simulink model "ModeAdjust"  (R2018b)
settings: Solver=FixedStepDiscrete  StartTime=0.0  StopTime=inf  FixedStep=0.01  RelTol=1e-3
undefined symbols (not defined in the file or in its folder): IfKeSMSbSeatMovBkRclnEnable_Val, IfKeSMSbSeatMovFrwdBkwdEnable_Val, IfKeSMSbSeatMovFtrstEnable_Val, IfKeSMSbSeatMovHdrstFrwdBkwdEnable_Val, IfKeSMSbSeatMovHdUpwdDnwdEnable_Val, IfKeSMSbSeatMovLgrstEnable_Val, IfKeSMSbSeatMovLtwdRtwdEnable_Val, IfVeSMSeStNumConfig, KeSMSbArmscreenMovEnable_Val, KeSMSbSeatMovLgrstExpdEnable_Val, KeSMSuFirstRwStBackPosDelta_Val, KeSMSuFirstRwStBackPosTolr_Val, KeSMSuFirstRwStCushFrntPosDelta_Val, KeSMSuFirstRwStCushFrntPosTolr_Val, KeSMSuFirstRwStCushRePosDelta_Val, KeSMSuFirstRwStCushRePosTolr_Val, KeSMSuFirstRwStFootrestPosDelta_Val, KeSMSuFirstRwStFootrestPosTolr_Val, KeSMSuFirstRwStFwdBkwdPosDelta_Val, KeSMSuFirstRwStFwdBkwdPosTolr_Val, KeSMSuMdMotFinshdTm_Val, KeSMSuMdRetryTm1_Val, KeSMSuModeReqDurgTm_Val, KeSMSuSecRwStArmTochPosDelta_Val, KeSMSuSecRwStArmTochPosTolr_Val, KeSMSuSecRwStBackPosDelta_Val, KeSMSuSecRwStBackPosTolr_Val, KeSMSuSecRwStFtrstUpwdDnwdPosDelta_Val, KeSMSuSecRwStFtrstUpwdDnwdPosTolr_Val, KeSMSuSecRwStFwdBkwdPosDelta_Val, KeSMSuSecRwStFwdBkwdPosTolr_Val, KeSMSuSecRwStHeadrestFwdBkwdPosDelta_Val, KeSMSuSecRwStHeadrestFwdBkwdPosTolr_Val, KeSMSuSecRwStHeadrestUpwdDwnwdPosDelta_Val, KeSMSuSecRwStHeadrestUpwdDwnwdPosTolr_Val, KeSMSuSecRwStLegrestInOutPosDelta_Val, KeSMSuSecRwStLegrestInOutPosTolr_Val, KeSMSuSecRwStLegrestUpwdDwnwdPosDelta_Val, KeSMSuSecRwStLegrestUpwdDwnwdPosTolr_Val, KeSMSuSecRwStLwdRwdPosDelta_Val, KeSMSuSecRwStLwdRwdPosTolr_Val, KeSMSuSecRwStVIPFtrstRefAngle_Val, KeSMSuThirdRwStFwdBkwdPosDelta_Val, KeSMSuThirdRwStFwdBkwdPosTolr_Val, KeSMSuThrdRwCushFoldPosDelta_Val, KeSMSuThrdRwCushFoldPosTolr_Val, KeSMSuThrdRwStBackPosDelta_Val, KeSMSuThrdRwStBackPosTolr_Val, KeSMSw4SLegrstCloseMdSecRwLtStFtrstUpwdDnwdPos_Val, KeSMSw4SLegrstCloseMdSecRwLtStFtrstUpwdDnwdPosMax_Val, KeSMSw4SLegrstCloseMdSecRwLtStFtrstUpwdDnwdPosMin_Val, KeSMSw4SLegrstCloseMdSecRwLtStLgrstOtwdInwdPos_Val, KeSMSw4SLegrstCloseMdSecRwLtStLgrstOtwdInwdPosMax_Val, KeSMSw4SLegrstCloseMdSecRwLtStLgrstOtwdInwdPosMin_Val, KeSMSw4SLegrstCloseMdSecRwLtStLgrstUpwdDnwdPos_Val, KeSMSw4SLegrstCloseMdSecRwLtStLgrstUpwdDnwdPosMax_Val, KeSMSw4SLegrstCloseMdSecRwLtStLgrstUpwdDnwdPosMin_Val, KeSMSw4SLegrstCloseMdSecRwRtStFtrstUpwdDnwdPos_Val, KeSMSw4SLegrstCloseMdSecRwRtStFtrstUpwdDnwdPosMax_Val, KeSMSw4SLegrstCloseMdSecRwRtStFtrstUpwdDnwdPosMin_Val ... (+1138)
libraries: Lib x401
(part 8 of 35)

== system ModeAdjust/ModeAdjustRunnable_sys/ModeAdjust/LgrstCloseR ==
  note: Change Request 179276
      | 复位模式头枕上下移动到第一步，第一步直接控制靠背、头枕上下、腿托系统同时运动，
      | 当腿托系统运动完成后进行头枕前后运动
  SecRwLtStsPoss : Inport
  SecRwLtStPossV : Inport  Port=2
  Recovery_Mod_Left : Inport  Port=3
  ModeStCalib : Inport  Port=4
  StConfig : Inport  Port=5
  SecRwLtStsPoss4s : Inport  Port=6
  SecRwLtStPossV4s : Inport  Port=7
  StConfig4s : Inport  Port=8
  isLfRecoveryArrivedAtTargetPos : Inport  Port=9
  Enable : EnablePort  StatesWhenEnabling=reset
  Bus Creator1 : BusCreator  Inputs=2
  Bus Selector : BusSelector  OutputSignals=Calib_Drv,Calib_Pass,Calib_2L,Calib_2R,Calib_3L,Calib_3R,Calib_2L4s,Calib_2R4s
  Bus Selector1 : BusSelector  OutputSignals=DrvStConfig,PassStConfig,SecRwLtStConfig,SecRwRtStConfig,ThdRwLtStConfig,ThdRwRtStConfig
  Bus Selector2 : BusSelector  OutputSignals=SecRwLtStConfig,SecRwRtStConfig
  Bus Selector3 : BusSelector  OutputSignals=IfVeSMSuSecRwRtStBkReclnUpwdDnwdPos_Val_read,IfVeSMSuSecRwRtStFrwdBkwdPos_Val_read,IfVeSMSuSecRwRtStHPassStUpwdDnwdPos_Val_read,IfVeSMSuSecRwRtStLgrstUpwdDnwdPos_Val_read,IfVeSMSuSecRwRtStLtwdRtwdPos_Val_read,SecRwRtStArmScrnPos_Val_read
  Bus Selector4 : BusSelector  OutputSignals=IfVeSMSuSecRwRtStBkReclnUpwdDnwdPosV_Val_read,IfVeSMSuSecRwRtStFrwdBkwdPosV_Val_read,IfVeSMSuSecRwRtStHPassStUpwdDnwdPosV_Val_read,IfVeSMSuSecRwRtStLgrstUpwdDnwdPosV_Val_read,IfVeSMSuSecRwRtStLtwdRtwdPosV_Val_read,SecRwRtStArmScrnPosV_Val_read
  Bus Selector5 : BusSelector  OutputSignals=IfVeSMSuSecRwRtStLgrstOtwdInwdPos_Val_read,IfVeSMSuRrRtStFtUpwdDnwdPos_Val_read,IfVeSMSuSecRwRtStHdrstFrwdBkwdPos_Val_read
  Bus Selector6 : BusSelector  OutputSignals=IfVeSMSuSecRwRtStLgrstOtwdInwdPosV_Val_read,IfVeSMSuRrRtStFtUpwdDnwdPosV_Val_read
  Chart : Stateflow chart  TreatAsAtomicUnit=on
  Chart1 : Stateflow chart  TreatAsAtomicUnit=on
  Logical Operator1 : Logic  Operator=NOT  AllPortsSameDT=off  OutDataTypeStr=boolean
  Logical Operator2 : Logic  Inputs=3  AllPortsSameDT=off  OutDataTypeStr=boolean
  Logical Operator3 : Logic  Operator=OR  AllPortsSameDT=off  OutDataTypeStr=boolean
  PA_KeSMSuSecRwStFtrstUpwdDnwdPosDelta_Val : Constant  Value=KeSMSuSecRwStFtrstUpwdDnwdPosDelta_Val
  PA_KeSMSuSecRwStLegrestInOutPosDelta_Val : Constant  Value=KeSMSuSecRwStLegrestInOutPosDelta_Val
  PA_KeSMSw4SSecRwLtStLgrstOtwdInwdClosePos1_Val : Constant  Value=KeSMSw4SSecRwLtStLgrstOtwdInwdClosePos1_Val
  PA_KeSMSw4SSecRwLtStLgrstUpwdDnwdClosePos1_Val : Constant  Value=KeSMSw4SSecRwLtStLgrstUpwdDnwdClosePos1_Val
  PA_KeSMSw4SSecRwLtStLgrstUpwdDnwdClosePos2_Val : Constant  Value=KeSMSw4SSecRwLtStLgrstUpwdDnwdClosePos2_Val
  R2Lt : Subsystem
  VIP_TrigJudg : Lib/VIP_TrigJudg  SystemSampleTime=-1
  R2Lt_TrgtPoss : Outport  VectorParamsAs1DForOutWhenUnconnected=on
  IfVeSMSuSecRwLtStRclCmdSrv_Val_writeRec : Outport  Port=2
  isAcsMdFeedBackNew_LyL : Outport  Port=3
  R2Lt_TrgtPoss_2 : Outport  Port=4  VectorParamsAs1DForOutWhenUnconnected=on
  wires:
  Logical Operator3/1 -> Chart1/1(Left_Done)
  R2Lt/2(IfVeSMSuSecRwLtStRclCmdSrv_Val_writeRaw) -> [IfVeSMSuSecRwLtStRclCmdSrv_Val_writeRaw]
  [IfVeSMSuSecRwLtStRclCmdSrv_Val_writeRaw] -> Chart1/2(IfVeSMSuSecRwLtStRclCmdSrv_Val_writeRaw)
  Recovery_Mod_Left/1 -> [Recovery_Mod_Left]
  VIP_TrigJudg/1 -> [EZE_TrigL]
  [EZE_TrigL] -> R2Lt/1(Mode_Trig)
  R2Lt/1(R2Lt_TrgtPoss) -> R2Lt_TrgtPoss/1
  SecRwLtStsPoss/1 -> R2Lt/2(SecRwLtStsPoss), [Pos]
  SecRwLtStPossV/1 -> R2Lt/3(SecRwLtStPossV), [PosV]
  [Recv_L_DoneOK] -> Chart1/3(Md_L_DoneOkRaw)
  [Recv_L_DoneFailed] -> Chart1/4(Md_L_DoneFailedRaw)
  Chart1/2(Md_L_DoneOk) -> [Ly_L_DoneOK]
  Chart1/3(Md_L_DoneFailed) -> [Ly_L_DoneFailed]
  Chart1/1(IfVeSMSuSecRwLtStRclCmdSrv_Val_write) -> IfVeSMSuSecRwLtStRclCmdSrv_Val_writeRec/1  "IfVeSMSuSecRwLtStRclCmdSrv_Val_write"
  Bus Selector/2 -> [ModeStCalib_Pass]  "<Calib_Pass>"
  Bus Selector/5 -> [ModeStCalib_3L]  "<Calib_3L>"
  Bus Selector/3 -> [ModeStCalib_2L]  "<Calib_2L>"
  Bus Selector/1 -> [ModeStCalib_Drv]  "<Calib_Drv>"
  Bus Selector/6 -> [ModeStCalib_3R]  "<Calib_3R>"
  Bus Selector/4 -> [ModeStCalib_2R]  "<Calib_2R>"
  ModeStCalib/1 -> Bus Selector/1
  [ModeStCalib_2R4s] -> R2Lt/4(ModeStCalib_2L)
  [Recovery_Mod_Left] -> VIP_TrigJudg/1
  Bus Creator1/1 -> isAcsMdFeedBackNew_LyL/1
  [Ly_L_DoneOK] -> Bus Creator1/1  "isLgrstCloseRDoneOK"
  [Ly_L_DoneFailed] -> Bus Creator1/2  "isLgrstCloseRDoneFailed"
  Bus Selector1/6 -> [ThdRwRtStConfig]  "<ThdRwRtStConfig>"
  Bus Selector1/1 -> [DrvStConfig]  "<DrvStConfig>"
  Bus Selector1/3 -> [SecRwLtStConfig]  "<SecRwLtStConfig>"
  Bus Selector1/4 -> [SecRwRtStConfig]  "<SecRwRtStConfig>"
  StConfig/1 -> Bus Selector1/1
  Bus Selector1/2 -> [PassStConfig]  "<PassStConfig>"
  Bus Selector1/5 -> [ThdRwLtStConfig]  "<ThdRwLtStConfig>"
  [SecRwLtStConfig] -> R2Lt/5(StConfig)
  Bus Selector/8 -> [ModeStCalib_2R4s]  "<Calib_2R4s>"
  Bus Selector/7 -> [ModeStCalib_2L4s]  "<Calib_2L4s>"
  SecRwLtStsPoss4s/1 -> [Pos4s], R2Lt/6(SecRwLtStsPoss4s)
  SecRwLtStPossV4s/1 -> R2Lt/7(SecRwLtStPossV4s), [PosV4s]
  StConfig4s/1 -> Bus Selector2/1
  Bus Selector2/1 -> [SecRwLtStConfig4s]  "<SecRwLtStConfig>"
  Bus Selector2/2 -> [SecRwRtStConfig4s]  "<SecRwRtStConfig>"
  [SecRwLtStConfig4s] -> R2Lt/8(StConfig4s)
  [PosV] -> Bus Selector4/1
  Bus Selector4/6 -> [R2LtStArmScrnPosV]  "<SecRwRtStArmScrnPosV_Val_read>"
  Bus Selector3/6 -> [R2LtStArmScrnPos]  "<SecRwRtStArmScrnPos_Val_read>"
  Bus Selector4/5 -> [SecRwLtStLtwdRtwdPosV]  "<IfVeSMSuSecRwRtStLtwdRtwdPosV_Val_read>"
  Bus Selector3/4 -> [SecRwLtStLgrstUpwdDnwdPos]  "<IfVeSMSuSecRwRtStLgrstUpwdDnwdPos_Val_read>"
  Bus Selector3/1 -> [SecRwLtStBkReclnUpwdDnwdPos]  "<IfVeSMSuSecRwRtStBkReclnUpwdDnwdPos_Val_read>"
  Bus Selector3/2 -> [SecRwLtStFrwdBkwdPos]  "<IfVeSMSuSecRwRtStFrwdBkwdPos_Val_read>"
  Bus Selector4/2 -> [SecRwLtStFrwdBkwdPosV]  "<IfVeSMSuSecRwRtStFrwdBkwdPosV_Val_read>"
  Bus Selector4/4 -> [SecRwLtStLgrstUpwdDnwdPosV]  "<IfVeSMSuSecRwRtStLgrstUpwdDnwdPosV_Val_read>"
  Bus Selector3/3 -> [SecRwLtStHPassStUpwdDnwdPos]  "<IfVeSMSuSecRwRtStHPassStUpwdDnwdPos_Val_read>"
  [Pos] -> Bus Selector3/1
  Bus Selector3/5 -> [SecRwLtStLtwdRtwdPos]  "<IfVeSMSuSecRwRtStLtwdRtwdPos_Val_read>"
  Bus Selector4/3 -> [SecRwLtStHPassStUpwdDnwdPosV]  "<IfVeSMSuSecRwRtStHPassStUpwdDnwdPosV_Val_read>"
  Bus Selector4/1 -> [SecRwLtStBkReclnUpwdDnwdPosV]  "<IfVeSMSuSecRwRtStBkReclnUpwdDnwdPosV_Val_read>"
  Bus Selector6/1 -> [SecRwLtStLgrstOtwdInwdPosV]  "<IfVeSMSuSecRwRtStLgrstOtwdInwdPosV_Val_read>"
  [Pos4s] -> Bus Selector5/1
  Bus Selector6/2 -> [RrLtStFtUpwdDnwdPosV]  "<IfVeSMSuRrRtStFtUpwdDnwdPosV_Val_read>"
  [PosV4s] -> Bus Selector6/1
  Bus Selector5/1 -> [SecRwLtStLgrstOtwdInwdPos]  "<IfVeSMSuSecRwRtStLgrstOtwdInwdPos_Val_read>"
  Bus Selector5/2 -> [RrLtStFtUpwdDnwdPos]  "<IfVeSMSuRrRtStFtUpwdDnwdPos_Val_read>"
  [SecRwLtStLgrstUpwdDnwdPos] -> Chart/1(downpos)
  [lgrstStep1_done] -> Chart/7(Step1done)
  [lgrstStep1_ini] -> Chart/10(Step1_ini)
  [lgrstStep2_ini] -> Chart/11(Step2_ini)
  [lgrstStep3_ini] -> Chart/12(Step3_ini)
  [lgrstStep2_done] -> Chart/8(Step2done)
  Chart/1(StepEn_LgrstStep1) -> [StepEn_LgrstStep1]
  Chart/2(StepEn_LgrstStep2) -> [StepEn_LgrstStep2]
  Chart/3(StepEn_LgrstStep3) -> [StepEn_LgrstStep3]
  R2Lt/9(R2Lt_TrgtPoss_2) -> R2Lt_TrgtPoss_2/1
  [lgrstStep3_done] -> Chart/9(Step3done)
  PA_KeSMSw4SSecRwLtStLgrstOtwdInwdClosePos1_Val/1 -> [CloseOtwdPos1]
  PA_KeSMSw4SSecRwLtStLgrstUpwdDnwdClosePos2_Val/1 -> [CloseDnwdPos2]
  PA_KeSMSw4SSecRwLtStLgrstUpwdDnwdClosePos1_Val/1 -> [CloseDnwdPos1]
  [CloseDnwdPos2] -> Chart/5(closedownpos2)
  [CloseDnwdPos1] -> Chart/4(closedownpos1)
  [CloseOtwdPos1] -> Chart/6(closeOtpos1)
  [RrLtStFtUpwdDnwdPos] -> Chart/3(Ftpos)
  [SecRwLtStLgrstOtwdInwdPos] -> Chart/2(Otpos)
  [StepEn_LgrstStep1] -> R2Lt/11(StepEn_LgrstStep3)
  [StepEn_LgrstStep3] -> R2Lt/10(StepEn_LgrstStep2)
  [StepEn_LgrstStep2] -> R2Lt/9(StepEn_LgrstStep1)
  PA_KeSMSuSecRwStFtrstUpwdDnwdPosDelta_Val/1 -> [KeSMSuSecRwStFtrstUpwdDnwdPosDelta_Val]
  [KeSMSuSecRwStFtrstUpwdDnwdPosDelta_Val] -> Chart/13(FtposDelta)
  R2Lt/6(lgrstStep1_done) -> [lgrstStep2_done]
  R2Lt/8(lgrstStep3_done) -> [lgrstStep1_done]
  R2Lt/7(lgrstStep2_done) -> [lgrstStep3_done]
  R2Lt/3(lgrstUpwd_ini) -> [lgrstStep2_ini]
  R2Lt/5(lgrstOtwd_ini) -> [lgrstStep1_ini]
  R2Lt/4(lgrstFtUpwd_ini) -> [lgrstStep3_ini]
  Logical Operator1/1 -> [Recv_L_DoneFailed]
  isLfRecoveryArrivedAtTargetPos/1 -> [Recv_L_DoneOK], Logical Operator1/1
  Bus Selector5/3 -> [SecRwLtStHdrstFrwdBkwdPos]  "<IfVeSMSuSecRwRtStHdrstFrwdBkwdPos_Val_read>"
  PA_KeSMSuSecRwStLegrestInOutPosDelta_Val/1 -> [KeSMSuSecRwStLegrestInOutPosDelta_Val]
  [KeSMSuSecRwStLegrestInOutPosDelta_Val] -> Chart/14(OtposDelta)
  Chart/4(failflg) -> [failflg]
  [lgrstStep3_done] -> Logical Operator2/3
  [lgrstStep2_done] -> Logical Operator2/2
  [lgrstStep1_done] -> Logical Operator2/1
  Logical Operator2/1 -> Logical Operator3/1
  [failflg] -> Logical Operator3/2

== system ModeAdjust/ModeAdjustRunnable_sys/ModeAdjust/LgrstOpenL ==
  SecRwLtStsPoss : Inport
  SecRwLtStPossV : Inport  Port=2
  Recovery_Mod_Left : Inport  Port=3
  ModeStCalib : Inport  Port=4
  StConfig : Inport  Port=5
  SecRwLtStsPoss4s : Inport  Port=6
  SecRwLtStPossV4s : Inport  Port=7
  StConfig4s : Inport  Port=8
  isLfVipArrivedAtTargetPos : Inport  Port=9
  Enable : EnablePort  StatesWhenEnabling=reset
  Bus Creator1 : BusCreator  Inputs=2
  Bus Selector : BusSelector  OutputSignals=Calib_Drv,Calib_Pass,Calib_2L,Calib_2R,Calib_3L,Calib_3R,Calib_2L4s,Calib_2R4s
  Bus Selector1 : BusSelector  OutputSignals=DrvStConfig,PassStConfig,SecRwLtStConfig,SecRwRtStConfig,ThdRwLtStConfig,ThdRwRtStConfig
  Bus Selector2 : BusSelector  OutputSignals=SecRwLtStConfig,SecRwRtStConfig
  Bus Selector3 : BusSelector  OutputSignals=IfVeSMSuSecRwLtStBkReclnUpwdDnwdPos_Val_read,IfVeSMSuSecRwLtStFrwdBkwdPos_Val_read,IfVeSMSuSecRwLtStHPassStUpwdDnwdPos_Val_read,IfVeSMSuSecRwLtStLgrstUpwdDnwdPos_Val_read,IfVeSMSuSecRwLtStLtwdRtwdPos_Val_read,IfVeSMSuSecRwLtStArmScrnPos_Val_read
  Bus Selector4 : BusSelector  OutputSignals=IfVeSMSuSecRwLtStBkReclnUpwdDnwdPosV_Val_read,IfVeSMSuSecRwLtStFrwdBkwdPosV_Val_read,IfVeSMSuSecRwLtStHPassStUpwdDnwdPosV_Val_read,IfVeSMSuSecRwLtStLgrstUpwdDnwdPosV_Val_read,IfVeSMSuSecRwLtStLtwdRtwdPosV_Val_read,IfVeSMSuSecRwLtStArmScrnPosV_Val_read
  Bus Selector5 : BusSelector  OutputSignals=IfVeSMSuSecRwLtStLgrstOtwdInwdPos_Val_read,IfVeSMSuRrLtStFtUpwdDnwdPos_Val_read,IfVeSMSuSecRwLtStHdrstFrwdBkwdPos_Val_read
  Bus Selector6 : BusSelector  OutputSignals=IfVeSMSuSecRwLtStLgrstOtwdInwdPosV_Val_read,IfVeSMSuRrLtStFtUpwdDnwdPosV_Val_read
  Chart : Stateflow chart  TreatAsAtomicUnit=on
  Chart1 : Stateflow chart  TreatAsAtomicUnit=on
  Logical Operator1 : Logic  Inputs=3  AllPortsSameDT=off  OutDataTypeStr=boolean
  Logical Operator2 : Logic  AllPortsSameDT=off  OutDataTypeStr=boolean
  Logical Operator3 : Logic  AllPortsSameDT=off  OutDataTypeStr=boolean
  Logical Operator4 : Logic  Operator=NOT  AllPortsSameDT=off  OutDataTypeStr=boolean
  Logical Operator{6..9} (4 alike) : Logic  Operator=OR  AllPortsSameDT=off  OutDataTypeStr=boolean
  PA_KeSMSw4SSecRwLtStLgrstUpwdDnwdOpenPos1_Val : Constant  Value=KeSMSw4SSecRwLtStLgrstUpwdDnwdOpenPos1_Val
  R2Lt : Subsystem
  Relational Operator : RelationalOperator  OutDataTypeStr=boolean  RndMeth=Simplest
  Unit Delay1 : UnitDelay  SampleTime=-1
  Unit Delay3 : UnitDelay  SampleTime=-1
  Unit Delay4 : UnitDelay  SampleTime=-1
  VIP_TrigJudg : Lib/VIP_TrigJudg  SystemSampleTime=-1
  R2Lt_TrgtPoss : Outport  VectorParamsAs1DForOutWhenUnconnected=on
  IfVeSMSuSecRwLtStRclCmdSrv_Val_write : Outport  Port=2
  isAcsMdFeedBackNew_LgrstOpenL : Outport  Port=3
  R2Lt_TrgtPoss_2 : Outport  Port=4  VectorParamsAs1DForOutWhenUnconnected=on
  wires:
  [lgrstStep3_ini] -> Logical Operator9/2
  [lgrstStep2_ini] -> Logical Operator8/2
  [lgrstStep1_ini] -> Logical Operator7/2
  [lgrstStep3_Chk] -> Logical Operator9/1
  [lgrstStep2_Chk] -> Logical Operator8/1
  [lgrstStep1_done] -> Logical Operator7/1
  Logical Operator7/1 -> Logical Operator1/1
  Logical Operator8/1 -> Logical Operator1/2
  Logical Operator9/1 -> Logical Operator1/3
  Bus Selector5/3 -> [SecRwLtStHdrstFrwdBkwdPos]  "<IfVeSMSuSecRwLtStHdrstFrwdBkwdPos_Val_read>"
  Logical Operator6/1 -> Chart1/1(Left_Done)
  Logical Operator1/1 -> Logical Operator6/1
  [failflg] -> Logical Operator6/2
  Chart/2(StepEn_LgrstStep2) -> [StepEn_LgrstStep2]
  Chart/3(StepEn_LgrstStep3) -> [StepEn_LgrstStep3]
  Chart/1(StepEn_LgrstStep1) -> [StepEn_LgrstStep1]
  Chart/4(failflg) -> [failflg]
  isLfVipArrivedAtTargetPos/1 -> Logical Operator4/1, [Recv_L_DoneOK]
  Logical Operator4/1 -> [Recv_L_DoneFailed]
  R2Lt/2(IfVeSMSuSecRwLtStRclCmdSrv_Val_writeRaw) -> [IfVeSMSuSecRwLtStRclCmdSrv_Val_writeRaw]
  [IfVeSMSuSecRwLtStRclCmdSrv_Val_writeRaw] -> Chart1/2(IfVeSMSuSecRwLtStRclCmdSrv_Val_writeRaw)
  Recovery_Mod_Left/1 -> [Recovery_Mod_Left]
  VIP_TrigJudg/1 -> [EZE_TrigL]
  [EZE_TrigL] -> R2Lt/1(Mode_Trig)
  R2Lt/1(R2Lt_TrgtPoss) -> R2Lt_TrgtPoss/1
  SecRwLtStsPoss/1 -> [Pos], R2Lt/2(SecRwLtStsPoss)
  SecRwLtStPossV/1 -> [PosV], R2Lt/3(SecRwLtStPossV)
  [Recv_L_DoneOK] -> Chart1/3(Md_L_DoneOkRaw)
  [Recv_L_DoneFailed] -> Chart1/4(Md_L_DoneFailedRaw)
  Chart1/2(Md_L_DoneOk) -> [Ly_L_DoneOK]
  Chart1/3(Md_L_DoneFailed) -> [Ly_L_DoneFailed]
  Chart1/1(IfVeSMSuSecRwLtStRclCmdSrv_Val_write) -> IfVeSMSuSecRwLtStRclCmdSrv_Val_write/1  "IfVeSMSuSecRwLtStRclCmdSrv_Val_write"
  Bus Selector/2 -> [ModeStCalib_Pass]  "<Calib_Pass>"
  Bus Selector/5 -> [ModeStCalib_3L]  "<Calib_3L>"
  Bus Selector/3 -> [ModeStCalib_2L]  "<Calib_2L>"
  Bus Selector/1 -> [ModeStCalib_Drv]  "<Calib_Drv>"
  Bus Selector/6 -> [ModeStCalib_3R]  "<Calib_3R>"
  Bus Selector/4 -> [ModeStCalib_2R]  "<Calib_2R>"
  ModeStCalib/1 -> Bus Selector/1
  [ModeStCalib_2L4s] -> R2Lt/4(ModeStCalib_2L)
  [Recovery_Mod_Left] -> VIP_TrigJudg/1
  Bus Creator1/1 -> isAcsMdFeedBackNew_LgrstOpenL/1
  [Ly_L_DoneOK] -> Bus Creator1/1  "isLgrstOpenLDoneOK"
  [Ly_L_DoneFailed] -> Bus Creator1/2  "isLgrstOpenLDoneFailed"
  Bus Selector1/6 -> [ThdRwRtStConfig]  "<ThdRwRtStConfig>"
  Bus Selector1/1 -> [DrvStConfig]  "<DrvStConfig>"
  Bus Selector1/3 -> [SecRwLtStConfig]  "<SecRwLtStConfig>"
  Bus Selector1/4 -> [SecRwRtStConfig]  "<SecRwRtStConfig>"
  StConfig/1 -> Bus Selector1/1
  Bus Selector1/2 -> [PassStConfig]  "<PassStConfig>"
  Bus Selector1/5 -> [ThdRwLtStConfig]  "<ThdRwLtStConfig>"
  [SecRwLtStConfig] -> R2Lt/5(StConfig)
  Bus Selector/8 -> [ModeStCalib_2R4s]  "<Calib_2R4s>"
  Bus Selector/7 -> [ModeStCalib_2L4s]  "<Calib_2L4s>"
  SecRwLtStsPoss4s/1 -> R2Lt/6(SecRwLtStsPoss4s), [Pos4s]
  SecRwLtStPossV4s/1 -> [PosV4s], R2Lt/7(SecRwLtStPossV4s)
  StConfig4s/1 -> Bus Selector2/1
  Bus Selector2/1 -> [SecRwLtStConfig4s]  "<SecRwLtStConfig>"
  Bus Selector2/2 -> [SecRwRtStConfig4s]  "<SecRwRtStConfig>"
  [SecRwLtStConfig4s] -> R2Lt/8(StConfig4s)
  [PosV] -> Bus Selector4/1
  Bus Selector4/6 -> [R2LtStArmScrnPosV]  "<IfVeSMSuSecRwLtStArmScrnPosV_Val_read>"
  Bus Selector3/6 -> [R2LtStArmScrnPos]  "<IfVeSMSuSecRwLtStArmScrnPos_Val_read>"
  Bus Selector4/5 -> [SecRwLtStLtwdRtwdPosV]  "<IfVeSMSuSecRwLtStLtwdRtwdPosV_Val_read>"
  Bus Selector3/4 -> [SecRwLtStLgrstUpwdDnwdPos]  "<IfVeSMSuSecRwLtStLgrstUpwdDnwdPos_Val_read>"
  Bus Selector3/1 -> [SecRwLtStBkReclnUpwdDnwdPos]  "<IfVeSMSuSecRwLtStBkReclnUpwdDnwdPos_Val_read>"
  Bus Selector3/2 -> [SecRwLtStFrwdBkwdPos]  "<IfVeSMSuSecRwLtStFrwdBkwdPos_Val_read>"
  Bus Selector4/2 -> [SecRwLtStFrwdBkwdPosV]  "<IfVeSMSuSecRwLtStFrwdBkwdPosV_Val_read>"
  Bus Selector4/4 -> [SecRwLtStLgrstUpwdDnwdPosV]  "<IfVeSMSuSecRwLtStLgrstUpwdDnwdPosV_Val_read>"
  Bus Selector3/3 -> [SecRwLtStHPassStUpwdDnwdPos]  "<IfVeSMSuSecRwLtStHPassStUpwdDnwdPos_Val_read>"
  [Pos] -> Bus Selector3/1
  Bus Selector3/5 -> [SecRwLtStLtwdRtwdPos]  "<IfVeSMSuSecRwLtStLtwdRtwdPos_Val_read>"
  Bus Selector4/3 -> [SecRwLtStHPassStUpwdDnwdPosV]  "<IfVeSMSuSecRwLtStHPassStUpwdDnwdPosV_Val_read>"
  Bus Selector4/1 -> [SecRwLtStBkReclnUpwdDnwdPosV]  "<IfVeSMSuSecRwLtStBkReclnUpwdDnwdPosV_Val_read>"
  Bus Selector6/1 -> [SecRwLtStLgrstOtwdInwdPosV]  "<IfVeSMSuSecRwLtStLgrstOtwdInwdPosV_Val_read>"
  [Pos4s] -> Bus Selector5/1
  Bus Selector6/2 -> [RrLtStFtUpwdDnwdPosV]  "<IfVeSMSuRrLtStFtUpwdDnwdPosV_Val_read>"
  [PosV4s] -> Bus Selector6/1
  Bus Selector5/1 -> [SecRwLtStLgrstOtwdInwdPos]  "<IfVeSMSuSecRwLtStLgrstOtwdInwdPos_Val_read>"
  Bus Selector5/2 -> [RrLtStFtUpwdDnwdPos]  "<IfVeSMSuRrLtStFtUpwdDnwdPos_Val_read>"
  [SecRwLtStLgrstUpwdDnwdPos] -> Chart/1(pos)
  [StepEn_LgrstStep1] -> R2Lt/9(StepEn_LgrstStep1)
  [StepEn_LgrstStep2] -> R2Lt/10(StepEn_LgrstStep2)
  [StepEn_LgrstStep3] -> R2Lt/11(StepEn_LgrstStep3)
  R2Lt/3(lgrstStep1_ini) -> [lgrstStep1_ini]
  R2Lt/5(lgrstStep3_ini) -> [lgrstStep3_ini]
  R2Lt/4(lgrstStep2_ini) -> [lgrstStep2_ini]
  R2Lt/6(lgrstStep1_done) -> [lgrstStep1_done]
  R2Lt/8(lgrstStep3_done) -> [lgrstStep3_done]
  R2Lt/7(lgrstStep2_done) -> [lgrstStep2_done]
  [lgrstStep1_done] -> Chart/3(Step1done)
  [lgrstStep1_ini] -> Chart/6(Step1_ini)
  [lgrstStep2_ini] -> Chart/7(Step2_ini)
  [lgrstStep3_ini] -> Chart/8(Step3_ini)
  PA_KeSMSw4SSecRwLtStLgrstUpwdDnwdOpenPos1_Val/1 -> [OpenPos1]
  [OpenPos1] -> Chart/2(openpos1)
  Logical Operator2/1 -> Unit Delay1/1
  [lgrstStep3_done] -> Logical Operator3/1
  [SecRwLtStLgrstUpwdDnwdPos] -> Relational Operator/1
  [OpenPos1] -> Relational Operator/2
  Relational Operator/1 -> Unit Delay3/1
  [lgrstStep2_done] -> Logical Operator2/2
  Unit Delay1/1 -> [lgrstStep2_Chk], Chart/4(Step2done)
  R2Lt/9(R2Lt_TrgtPoss_2) -> R2Lt_TrgtPoss_2/1
  Unit Delay3/1 -> Logical Operator2/1
  [lgrstStep2_Chk] -> Unit Delay4/1
  Logical Operator3/1 -> Chart/5(Step3done), [lgrstStep3_Chk]
  Unit Delay4/1 -> Logical Operator3/2

== system ModeAdjust/ModeAdjustRunnable_sys/ModeAdjust/LgrstOpenR ==
  SecRwLtStsPoss : Inport
  SecRwLtStPossV : Inport  Port=2
  Recovery_Mod_Left : Inport  Port=3
  ModeStCalib : Inport  Port=4
  StConfig : Inport  Port=5
  SecRwLtStsPoss4s : Inport  Port=6
  SecRwLtStPossV4s : Inport  Port=7
  StConfig4s : Inport  Port=8
  isLfVipArrivedAtTargetPos : Inport  Port=9
  Enable : EnablePort  StatesWhenEnabling=reset
  Bus Creator1 : BusCreator  Inputs=2
  Bus Selector : BusSelector  OutputSignals=Calib_Drv,Calib_Pass,Calib_2L,Calib_2R,Calib_3L,Calib_3R,Calib_2L4s,Calib_2R4s
  Bus Selector1 : BusSelector  OutputSignals=DrvStConfig,PassStConfig,SecRwLtStConfig,SecRwRtStConfig,ThdRwLtStConfig,ThdRwRtStConfig
  Bus Selector2 : BusSelector  OutputSignals=SecRwLtStConfig,SecRwRtStConfig
  Bus Selector3 : BusSelector  OutputSignals=IfVeSMSuSecRwRtStBkReclnUpwdDnwdPos_Val_read,IfVeSMSuSecRwRtStFrwdBkwdPos_Val_read,IfVeSMSuSecRwRtStHPassStUpwdDnwdPos_Val_read,IfVeSMSuSecRwRtStLgrstUpwdDnwdPos_Val_read,IfVeSMSuSecRwRtStLtwdRtwdPos_Val_read,SecRwRtStArmScrnPos_Val_read
  Bus Selector4 : BusSelector  OutputSignals=IfVeSMSuSecRwRtStBkReclnUpwdDnwdPosV_Val_read,IfVeSMSuSecRwRtStFrwdBkwdPosV_Val_read,IfVeSMSuSecRwRtStHPassStUpwdDnwdPosV_Val_read,IfVeSMSuSecRwRtStLgrstUpwdDnwdPosV_Val_read,IfVeSMSuSecRwRtStLtwdRtwdPosV_Val_read,SecRwRtStArmScrnPosV_Val_read
  Bus Selector5 : BusSelector  OutputSignals=IfVeSMSuSecRwRtStLgrstOtwdInwdPos_Val_read,IfVeSMSuRrRtStFtUpwdDnwdPos_Val_read,IfVeSMSuSecRwRtStHdrstFrwdBkwdPos_Val_read
  Bus Selector6 : BusSelector  OutputSignals=IfVeSMSuSecRwRtStLgrstOtwdInwdPosV_Val_read,IfVeSMSuRrRtStFtUpwdDnwdPosV_Val_read
  Chart : Stateflow chart  TreatAsAtomicUnit=on
  Chart1 : Stateflow chart  TreatAsAtomicUnit=on
  Logical Operator1 : Logic  Inputs=3  AllPortsSameDT=off  OutDataTypeStr=boolean
  Logical Operator2 : Logic  AllPortsSameDT=off  OutDataTypeStr=boolean
  Logical Operator3 : Logic  AllPortsSameDT=off  OutDataTypeStr=boolean
  Logical Operator4 : Logic  Operator=NOT  AllPortsSameDT=off  OutDataTypeStr=boolean
  Logical Operator{6..9} (4 alike) : Logic  Operator=OR  AllPortsSameDT=off  OutDataTypeStr=boolean
  PA_KeSMSw4SSecRwLtStLgrstUpwdDnwdOpenPos1_Val : Constant  Value=KeSMSw4SSecRwLtStLgrstUpwdDnwdOpenPos1_Val
  R2Lt : Subsystem
  Relational Operator : RelationalOperator  OutDataTypeStr=boolean  RndMeth=Simplest
  Unit Delay1 : UnitDelay  SampleTime=-1
  Unit Delay3 : UnitDelay  SampleTime=-1
  Unit Delay4 : UnitDelay  SampleTime=-1
  VIP_TrigJudg : Lib/VIP_TrigJudg  SystemSampleTime=-1
  R2Lt_TrgtPoss : Outport  VectorParamsAs1DForOutWhenUnconnected=on
  IfVeSMSuSecRwLtStRclCmdSrv_Val_writeRec : Outport  Port=2
  isAcsMdFeedBackNew_LgrstOpenL : Outport  Port=3
  R2Lt_TrgtPoss_2 : Outport  Port=4  VectorParamsAs1DForOutWhenUnconnected=on
  wires:
  Unit Delay4/1 -> Logical Operator3/2
  Logical Operator3/1 -> Chart/5(Step3done), [lgrstStep3_Chk]
  [lgrstStep2_Chk] -> Unit Delay4/1
  Unit Delay3/1 -> Logical Operator2/1
  R2Lt/9(R2Rt_TrgtPoss_2) -> R2Lt_TrgtPoss_2/1
  Unit Delay1/1 -> Chart/4(Step2done), [lgrstStep2_Chk]
  [lgrstStep2_done] -> Logical Operator2/2
  Relational Operator/1 -> Unit Delay3/1
  [OpenPos1] -> Relational Operator/2
  [SecRwLtStLgrstUpwdDnwdPos] -> Relational Operator/1
  [lgrstStep3_done] -> Logical Operator3/1
  Logical Operator2/1 -> Unit Delay1/1
  [OpenPos1] -> Chart/2(openpos1)
  PA_KeSMSw4SSecRwLtStLgrstUpwdDnwdOpenPos1_Val/1 -> [OpenPos1]
  [lgrstStep3_ini] -> Chart/8(Step3_ini)
  [lgrstStep2_ini] -> Chart/7(Step2_ini)
  [lgrstStep1_ini] -> Chart/6(Step1_ini)
  [lgrstStep1_done] -> Chart/3(Step1done)
  R2Lt/7(lgrstStep2_done) -> [lgrstStep2_done]
  R2Lt/8(lgrstStep3_done) -> [lgrstStep3_done]
  R2Lt/6(lgrstStep1_done) -> [lgrstStep1_done]
  R2Lt/4(lgrstStep2_ini) -> [lgrstStep2_ini]
  R2Lt/5(lgrstStep3_ini) -> [lgrstStep3_ini]
  R2Lt/3(lgrstStep1_ini) -> [lgrstStep1_ini]
  [StepEn_LgrstStep3] -> R2Lt/11(StepEn_LgrstStep3)
  [StepEn_LgrstStep2] -> R2Lt/10(StepEn_LgrstStep2)
  [StepEn_LgrstStep1] -> R2Lt/9(StepEn_LgrstStep1)
  [SecRwLtStLgrstUpwdDnwdPos] -> Chart/1(pos)
  Bus Selector5/2 -> [RrLtStFtUpwdDnwdPos]  "<IfVeSMSuRrRtStFtUpwdDnwdPos_Val_read>"
  Bus Selector5/1 -> [SecRwLtStLgrstOtwdInwdPos]  "<IfVeSMSuSecRwRtStLgrstOtwdInwdPos_Val_read>"
  [PosV4s] -> Bus Selector6/1
  Bus Selector6/2 -> [RrLtStFtUpwdDnwdPosV]  "<IfVeSMSuRrRtStFtUpwdDnwdPosV_Val_read>"
  [Pos4s] -> Bus Selector5/1
  Bus Selector6/1 -> [SecRwLtStLgrstOtwdInwdPosV]  "<IfVeSMSuSecRwRtStLgrstOtwdInwdPosV_Val_read>"
  Bus Selector4/1 -> [SecRwLtStBkReclnUpwdDnwdPosV]  "<IfVeSMSuSecRwRtStBkReclnUpwdDnwdPosV_Val_read>"
  Bus Selector4/3 -> [SecRwLtStHPassStUpwdDnwdPosV]  "<IfVeSMSuSecRwRtStHPassStUpwdDnwdPosV_Val_read>"
  Bus Selector3/5 -> [SecRwLtStLtwdRtwdPos]  "<IfVeSMSuSecRwRtStLtwdRtwdPos_Val_read>"
  [Pos] -> Bus Selector3/1
  Bus Selector3/3 -> [SecRwLtStHPassStUpwdDnwdPos]  "<IfVeSMSuSecRwRtStHPassStUpwdDnwdPos_Val_read>"
  Bus Selector4/4 -> [SecRwLtStLgrstUpwdDnwdPosV]  "<IfVeSMSuSecRwRtStLgrstUpwdDnwdPosV_Val_read>"
  Bus Selector4/2 -> [SecRwLtStFrwdBkwdPosV]  "<IfVeSMSuSecRwRtStFrwdBkwdPosV_Val_read>"
  Bus Selector3/2 -> [SecRwLtStFrwdBkwdPos]  "<IfVeSMSuSecRwRtStFrwdBkwdPos_Val_read>"
  Bus Selector3/1 -> [SecRwLtStBkReclnUpwdDnwdPos]  "<IfVeSMSuSecRwRtStBkReclnUpwdDnwdPos_Val_read>"
  Bus Selector3/4 -> [SecRwLtStLgrstUpwdDnwdPos]  "<IfVeSMSuSecRwRtStLgrstUpwdDnwdPos_Val_read>"
  Bus Selector4/5 -> [SecRwLtStLtwdRtwdPosV]  "<IfVeSMSuSecRwRtStLtwdRtwdPosV_Val_read>"
  Bus Selector3/6 -> [R2LtStArmScrnPos]  "<SecRwRtStArmScrnPos_Val_read>"
  Bus Selector4/6 -> [R2LtStArmScrnPosV]  "<SecRwRtStArmScrnPosV_Val_read>"
  [PosV] -> Bus Selector4/1
  [SecRwLtStConfig4s] -> R2Lt/8(StConfig4s)
  Bus Selector2/2 -> [SecRwRtStConfig4s]  "<SecRwRtStConfig>"
  Bus Selector2/1 -> [SecRwLtStConfig4s]  "<SecRwLtStConfig>"
  StConfig4s/1 -> Bus Selector2/1
  SecRwLtStPossV4s/1 -> R2Lt/7(SecRwLtStPossV4s), [PosV4s]
  SecRwLtStsPoss4s/1 -> [Pos4s], R2Lt/6(SecRwLtStsPoss4s)
  Bus Selector/7 -> [ModeStCalib_2L4s]  "<Calib_2L4s>"
  Bus Selector/8 -> [ModeStCalib_2R4s]  "<Calib_2R4s>"
  [SecRwLtStConfig] -> R2Lt/5(StConfig)
  Bus Selector1/5 -> [ThdRwLtStConfig]  "<ThdRwLtStConfig>"
  Bus Selector1/2 -> [PassStConfig]  "<PassStConfig>"
  StConfig/1 -> Bus Selector1/1
  Bus Selector1/4 -> [SecRwRtStConfig]  "<SecRwRtStConfig>"
  Bus Selector1/3 -> [SecRwLtStConfig]  "<SecRwLtStConfig>"
  Bus Selector1/1 -> [DrvStConfig]  "<DrvStConfig>"
  Bus Selector1/6 -> [ThdRwRtStConfig]  "<ThdRwRtStConfig>"
  [Ly_L_DoneFailed] -> Bus Creator1/2  "isLgrstOpenRDoneFailed"
  [Ly_L_DoneOK] -> Bus Creator1/1  "isLgrstOpenRDoneOK"
  Bus Creator1/1 -> isAcsMdFeedBackNew_LgrstOpenL/1
  [Recovery_Mod_Left] -> VIP_TrigJudg/1
  [ModeStCalib_2R4s] -> R2Lt/4(ModeStCalib_2L)
  ModeStCalib/1 -> Bus Selector/1
  Bus Selector/4 -> [ModeStCalib_2R]  "<Calib_2R>"
  Bus Selector/6 -> [ModeStCalib_3R]  "<Calib_3R>"
  Bus Selector/1 -> [ModeStCalib_Drv]  "<Calib_Drv>"
  Bus Selector/3 -> [ModeStCalib_2L]  "<Calib_2L>"
  Bus Selector/5 -> [ModeStCalib_3L]  "<Calib_3L>"
  Bus Selector/2 -> [ModeStCalib_Pass]  "<Calib_Pass>"
  Chart1/1(IfVeSMSuSecRwLtStRclCmdSrv_Val_write) -> IfVeSMSuSecRwLtStRclCmdSrv_Val_writeRec/1  "IfVeSMSuSecRwLtStRclCmdSrv_Val_write"
  Chart1/3(Md_L_DoneFailed) -> [Ly_L_DoneFailed]
  Chart1/2(Md_L_DoneOk) -> [Ly_L_DoneOK]
  [Recv_L_DoneFailed] -> Chart1/4(Md_L_DoneFailedRaw)
  [Recv_L_DoneOK] -> Chart1/3(Md_L_DoneOkRaw)
  SecRwLtStPossV/1 -> R2Lt/3(SecRwLtStPossV), [PosV]
  SecRwLtStsPoss/1 -> R2Lt/2(SecRwLtStsPoss), [Pos]
  R2Lt/1(R2Rt_TrgtPoss) -> R2Lt_TrgtPoss/1
  [EZE_TrigL] -> R2Lt/1(Mode_Trig)
  VIP_TrigJudg/1 -> [EZE_TrigL]
  Recovery_Mod_Left/1 -> [Recovery_Mod_Left]
  [IfVeSMSuSecRwLtStRclCmdSrv_Val_writeRaw] -> Chart1/2(IfVeSMSuSecRwLtStRclCmdSrv_Val_writeRaw)
  R2Lt/2(IfVeSMSuSecRwLtStRclCmdSrv_Val_writeRaw) -> [IfVeSMSuSecRwLtStRclCmdSrv_Val_writeRaw]
  Logical Operator4/1 -> [Recv_L_DoneFailed]
  isLfVipArrivedAtTargetPos/1 -> [Recv_L_DoneOK], Logical Operator4/1
  Chart/4(failflg) -> [failflg]
  Chart/1(StepEn_LgrstStep1) -> [StepEn_LgrstStep1]
  Chart/3(StepEn_LgrstStep3) -> [StepEn_LgrstStep3]
  Chart/2(StepEn_LgrstStep2) -> [StepEn_LgrstStep2]
  [failflg] -> Logical Operator6/2
  Logical Operator1/1 -> Logical Operator6/1
  Logical Operator6/1 -> Chart1/1(Left_Done)
  Bus Selector5/3 -> [SecRwLtStHdrstFrwdBkwdPos]  "<IfVeSMSuSecRwRtStHdrstFrwdBkwdPos_Val_read>"
  Logical Operator9/1 -> Logical Operator1/3
  Logical Operator8/1 -> Logical Operator1/2
  Logical Operator7/1 -> Logical Operator1/1
  [lgrstStep1_done] -> Logical Operator7/1
  [lgrstStep2_Chk] -> Logical Operator8/1
  [lgrstStep3_Chk] -> Logical Operator9/1
  [lgrstStep1_ini] -> Logical Operator7/2
  [lgrstStep2_ini] -> Logical Operator8/2
  [lgrstStep3_ini] -> Logical Operator9/2

== system ModeAdjust/ModeAdjustRunnable_sys/ModeAdjust/LugL ==
  ThdRwLtStPoss : Inport
  ThdRwLtStPossV : Inport  Port=2
  isR3Occupied : Inport  Port=3
  Lug_Mod_Left : Inport  Port=4
  ModeStCalib : Inport  Port=5
  is6s : Inport  Port=6
  StConfig : Inport  Port=7
  isLfLugArrivedAtTargetPos : Inport  Port=8
  ThdRwLtStFrwdCmdSrv : Inport  Port=9
  Enable : EnablePort  StatesWhenEnabling=reset
  Bus Creator1 : BusCreator  Inputs=2
  Bus Selector : BusSelector  OutputSignals=Calib_Drv,Calib_Pass,Calib_2L,Calib_2R,Calib_3L,Calib_3R
  Bus Selector1 : BusSelector  OutputSignals=DrvStConfig,PassStConfig,SecRwLtStConfig,SecRwRtStConfig,ThdRwLtStConfig,ThdRwRtStConfig
  Chart : Stateflow chart  TreatAsAtomicUnit=on
  Chart1 : Stateflow chart  TreatAsAtomicUnit=on
  Logical Operator : Logic  Operator=NOT  AllPortsSameDT=off  OutDataTypeStr=boolean
  R3Lt : Subsystem
  Terminator{,1..4} (5 alike) : Terminator
  VIP_TrigJudg : Lib/VIP_TrigJudg  SystemSampleTime=-1
  R3Lt_TrgtPoss : Outport  VectorParamsAs1DForOutWhenUnconnected=on
  IfVeSMSbThdRwLtStRclCmdSrv_Val_writeLug : Outport  Port=2
  isAcsMdFeedBackNew_LugL : Outport  Port=3
  LugLDone : Outport  Port=4
  R3Lt_SpdCtrl : Outport  Port=5  VectorParamsAs1DForOutWhenUnconnected=on
  wires:
  isR3Occupied/1 -> R3Lt/4(isSeatOccupied)
  ThdRwLtStPossV/1 -> R3Lt/6(ThdRwLtStPossV)
  ThdRwLtStPoss/1 -> R3Lt/5(ThdRwLtStPoss)
  [EZE_TrigL] -> R3Lt/1(Mode_Trig)
  R3Lt/6(R3Lt_TrgtPoss) -> R3Lt_TrgtPoss/1
  [IfVeSMSbThdRwLtStRclCmdSrv_Val_writeRaw] -> Chart1/2(IfVeSMSbThdRwLtStRclCmdSrv_Val_writeRaw)
  R3Lt/5(IfVeSMSbThdRwLtStRclCmdSrv_Val_writeRaw) -> [IfVeSMSbThdRwLtStRclCmdSrv_Val_writeRaw]
  R3Lt/4(R3Lt_Step2done) -> [R3Lt_Step2_done]
  R3Lt/1(R3Lt_Step1_ini) -> [R3Lt_Step1_ini]
  VIP_TrigJudg/1 -> [EZE_TrigL]
  R3Lt/2(R3Lt_Step2_ini) -> [R3Lt_Step2_ini]
  R3Lt/3(R3Lt_Step1done) -> [R3Lt_Step1_done]
  [R3Lt_All_done_1] -> LugLDone/1, Chart1/1(Left_Done)
  Lug_Mod_Left/1 -> [Lug_Mod_Left]
  [R3Lt_Step1_ini] -> Chart/1(R3Lt_Step1_ini)
  [R3Lt_Step2_ini] -> Chart/2(R3Lt_Step2_ini)
  [R3Lt_Step1_done] -> Chart/3(R3Lt_Step1_done)
  [R3Lt_Step2_done] -> Chart/4(R3Lt_Step2_done)
  Chart/1(R3Lt_Step1En) -> [R3Lt_Step1En]
  [R3Lt_Step1En] -> R3Lt/2(Step1En)
  [R3Lt_Step2En] -> R3Lt/3(Step2En)
  Chart/2(R3Lt_Step2En) -> [R3Lt_Step2En]
  [Md_L_MvDoneOK] -> Chart1/3(Md_L_DoneOkRaw)
  [Md_L_MvDoneFailed] -> Chart1/4(Md_L_DoneFailedRaw)
  Chart1/2(Md_L_DoneOk) -> [Lug_L_MvDoneOK]
  Chart1/3(Md_L_DoneFailed) -> [Lug_L_MvDoneFailed]
  Chart1/1(IfVeSMSbThdRwLtStRclCmdSrv_Val_write) -> IfVeSMSbThdRwLtStRclCmdSrv_Val_writeLug/1  "IfVeSMSbThdRwLtStRclCmdSrv_Val_write"
  R3Lt/7(R3Lt_All_done) -> [R3Lt_All_done_1]
  Bus Selector/2 -> Terminator1/1  "<Calib_Pass>"
  Bus Selector/5 -> [ModeStCalib_3L]  "<Calib_3L>"
  Bus Selector/3 -> Terminator2/1  "<Calib_2L>"
  Bus Selector/1 -> Terminator/1  "<Calib_Drv>"
  Bus Selector/6 -> Terminator4/1  "<Calib_3R>"
  Bus Selector/4 -> Terminator3/1  "<Calib_2R>"
  ModeStCalib/1 -> Bus Selector/1
  [ModeStCalib_3L] -> R3Lt/7(ModeStCalib_3L)
  is6s/1 -> [is6s]
  [is6s] -> R3Lt/8(is6s)
  [Lug_Mod_Left] -> VIP_TrigJudg/1
  Bus Creator1/1 -> isAcsMdFeedBackNew_LugL/1
  [Lug_L_MvDoneOK] -> Bus Creator1/1  "isLfLugDoneOK"
  [Lug_L_MvDoneFailed] -> Bus Creator1/2  "isLfLugDoneFailed"
  Bus Selector1/6 -> [ThdRwRtStConfig]  "<ThdRwRtStConfig>"
  Bus Selector1/1 -> [DrvStConfig]  "<DrvStConfig>"
  Bus Selector1/3 -> [SecRwLtStConfig]  "<SecRwLtStConfig>"
  Bus Selector1/4 -> [SecRwRtStConfig]  "<SecRwRtStConfig>"
  StConfig/1 -> Bus Selector1/1
  Bus Selector1/2 -> [PassStConfig]  "<PassStConfig>"
  Bus Selector1/5 -> [ThdRwLtStConfig]  "<ThdRwLtStConfig>"
  [ThdRwLtStConfig] -> R3Lt/9(StConfig)
  Logical Operator/1 -> [Md_L_MvDoneFailed]
  isLfLugArrivedAtTargetPos/1 -> [Md_L_MvDoneOK], Logical Operator/1
  R3Lt/8(R3Lt_SpdCtrl) -> R3Lt_SpdCtrl/1
  ThdRwLtStFrwdCmdSrv/1 -> R3Lt/10(ThdRwLtStFrwdCmdSrv)

== system ModeAdjust/ModeAdjustRunnable_sys/ModeAdjust/LugR ==
  ThdRwRtStPoss : Inport
  ThdRwRtStPossV : Inport  Port=2
  isR3RtSeatOccupied : Inport  Port=3
  Lug_Mod_Right : Inport  Port=4
  ModeStCalib : Inport  Port=5
  is6s : Inport  Port=6
  StConfig : Inport  Port=7
  isRtLugArrivedAtTargetPos : Inport  Port=8
  ThdRwRtStFrwdCmdSrv : Inport  Port=9
  Enable : EnablePort  StatesWhenEnabling=reset
  Bus Creator2 : BusCreator  Inputs=2
  Bus Selector : BusSelector  OutputSignals=Calib_Drv,Calib_Pass,Calib_2L,Calib_2R,Calib_3L,Calib_3R
  Bus Selector1 : BusSelector  OutputSignals=DrvStConfig,PassStConfig,SecRwLtStConfig,SecRwRtStConfig,ThdRwLtStConfig,ThdRwRtStConfig
  Chart : Stateflow chart  TreatAsAtomicUnit=on
  Chart1 : Stateflow chart  TreatAsAtomicUnit=on
  Logical Operator : Logic  Operator=NOT  AllPortsSameDT=off  OutDataTypeStr=boolean
  R3Rt : Subsystem
  VIP_TrigJudg1 : Lib/VIP_TrigJudg  SystemSampleTime=-1
  R3Rt_TrgtPoss : Outport  VectorParamsAs1DForOutWhenUnconnected=on
  IfVeSMSbThdRwRtStRclCmdSrv_Val_writeLug : Outport  Port=2
  isAcsMdFeedBackNew_LugR : Outport  Port=3
  LugRDone : Outport  Port=4
  R3Rt_SpdCtrl : Outport  Port=5  VectorParamsAs1DForOutWhenUnconnected=on
  wires:
  [Lug_R_MvDoneFailed] -> Bus Creator2/2  "isRtLugDoneFailed"
  [Lug_R_MvDoneOK] -> Bus Creator2/1  "isRtLugDoneOK"
  Bus Creator2/1 -> isAcsMdFeedBackNew_LugR/1
  [R3Lt_All_done_2] -> LugRDone/1, Chart1/1(Right_Done)
  VIP_TrigJudg1/1 -> [EZE_TrigR]
  [Lug_Mod_Right] -> VIP_TrigJudg1/1
  [is6s] -> R3Rt/8(is6s)
  is6s/1 -> [is6s]
  [ModeStCalib_3R] -> R3Rt/7(ModeStCalib_3R)
  ModeStCalib/1 -> Bus Selector/1
  Bus Selector/4 -> [ModeStCalib_2R]  "<Calib_2R>"
  Bus Selector/6 -> [ModeStCalib_3R]  "<Calib_3R>"
  Bus Selector/1 -> [ModeStCalib_Drv]  "<Calib_Drv>"
  Bus Selector/3 -> [ModeStCalib_2L]  "<Calib_2L>"
  Bus Selector/5 -> [ModeStCalib_3L]  "<Calib_3L>"
  Bus Selector/2 -> [ModeStCalib_Pass]  "<Calib_Pass>"
  R3Rt/7(R3Rt_All_done) -> [R3Lt_All_done_2]
  Chart1/1(IfVeSMSbThdRwRtStRclCmdSrv_Val_write) -> IfVeSMSbThdRwRtStRclCmdSrv_Val_writeLug/1  "IfVeSMSbThdRwRtStRclCmdSrv_Val_write"
  Chart1/3(Md_R_DoneFailed) -> [Lug_R_MvDoneFailed]
  Chart1/2(Md_R_DoneOk) -> [Lug_R_MvDoneOK]
  [Md_R_MvDoneOK] -> Chart1/3(Md_R_DoneOkRaw)
  [R3Rt_Step2En] -> R3Rt/3(Step2En)
  [R3Rt_Step1En] -> R3Rt/2(Step1En)
  Chart/2(R3Rt_Step2En) -> [R3Rt_Step2En]
  Chart/1(R3Rt_Step1En) -> [R3Rt_Step1En]
  [R3Rt_Step2_done] -> Chart/4(R3Rt_Step2_done)
  [R3Rt_Step1_done] -> Chart/3(R3Rt_Step1_done)
  [R3Rt_Step2_ini] -> Chart/2(R3Rt_Step2_ini)
  [R3Rt_Step1_ini] -> Chart/1(R3Rt_Step1_ini)
  Lug_Mod_Right/1 -> [Lug_Mod_Right]
  [EZE_TrigR] -> R3Rt/1(Mode_Trig)
  R3Rt/1(R3Rt_Step1_ini) -> [R3Rt_Step1_ini]
  R3Rt/2(R3Rt_Step2_ini) -> [R3Rt_Step2_ini]
  R3Rt/3(R3Rt_Step1done) -> [R3Rt_Step1_done]
  R3Rt/4(R3Rt_Step2_done) -> [R3Rt_Step2_done]
  R3Rt/5(IfVeSMSbThdRwRtStRclCmdSrv_Val_writeRaw) -> [IfVeSMSbThdRwRtStRclCmdSrv_Val_writeRaw]
  [IfVeSMSbThdRwRtStRclCmdSrv_Val_writeRaw] -> Chart1/2(IfVeSMSbThdRwRtStRclCmdSrv_Val_writeRaw)
  R3Rt/6(R3Rt_TrgtPoss) -> R3Rt_TrgtPoss/1
  ThdRwRtStPoss/1 -> R3Rt/5(ThdRwRtStPoss)
  ThdRwRtStPossV/1 -> R3Rt/6(ThdRwRtStPossV)
  isR3RtSeatOccupied/1 -> R3Rt/4(SeatOccupied)
  Bus Selector1/4 -> [SecRwRtStConfig]  "<SecRwRtStConfig>"
  Bus Selector1/6 -> [ThdRwRtStConfig]  "<ThdRwRtStConfig>"
  Bus Selector1/2 -> [PassStConfig]  "<PassStConfig>"
  Bus Selector1/3 -> [SecRwLtStConfig]  "<SecRwLtStConfig>"
  StConfig/1 -> Bus Selector1/1
  Bus Selector1/5 -> [ThdRwLtStConfig]  "<ThdRwLtStConfig>"
  Bus Selector1/1 -> [DrvStConfig]  "<DrvStConfig>"
  [ThdRwRtStConfig] -> R3Rt/9(StConfig)
  [Md_R_MvDoneFailed] -> Chart1/4(Md_R_DoneFailedRaw)
  Logical Operator/1 -> [Md_R_MvDoneFailed]
  isRtLugArrivedAtTargetPos/1 -> Logical Operator/1, [Md_R_MvDoneOK]
  R3Rt/8(R3Lt_SpdCtrl) -> R3Rt_SpdCtrl/1
  ThdRwRtStFrwdCmdSrv/1 -> R3Rt/10(ThdRwRtStFrwdCmdSrv)

== system ModeAdjust/ModeAdjustRunnable_sys/ModeAdjust/LyL ==
  SecRwLtStsPoss : Inport
  SecRwLtStPossV : Inport  Port=2
  SecRwRtStChldLkRsp_L : Inport  Port=3
  Recovery_Mod_Left : Inport  Port=4
  ModeStCalib : Inport  Port=5
  StConfig : Inport  Port=6
  SecRwLtStsPoss4s : Inport  Port=7
  SecRwLtStPossV4s : Inport  Port=8
  StConfig4s : Inport  Port=9
  isLfLyArrivedAtTargetPos : Inport  Port=10
  Calib_Ly4sLAdpt : Inport  Port=11
  Enable : EnablePort  StatesWhenEnabling=reset
  Bus Creator1 : BusCreator  Inputs=2
  Bus Selector : BusSelector  OutputSignals=Calib_Drv,Calib_Pass,Calib_2L,Calib_2R,Calib_3L,Calib_3R,Calib_2L4s,Calib_2R4s
  Bus Selector1 : BusSelector  OutputSignals=DrvStConfig,PassStConfig,SecRwLtStConfig,SecRwRtStConfig,ThdRwLtStConfig,ThdRwRtStConfig
  Bus Selector2 : BusSelector  OutputSignals=SecRwLtStConfig,SecRwRtStConfig
  Bus Selector3 : BusSelector  OutputSignals=IfVeSMSuSecRwLtStBkReclnUpwdDnwdPos_Val_read,IfVeSMSuSecRwLtStFrwdBkwdPos_Val_read,IfVeSMSuSecRwLtStHPassStUpwdDnwdPos_Val_read,IfVeSMSuSecRwLtStLgrstUpwdDnwdPos_Val_read,IfVeSMSuSecRwLtStLtwdRtwdPos_Val_read,IfVeSMSuSecRwLtStArmScrnPos_Val_read
  Bus Selector4 : BusSelector  OutputSignals=IfVeSMSuSecRwLtStBkReclnUpwdDnwdPosV_Val_read,IfVeSMSuSecRwLtStFrwdBkwdPosV_Val_read,IfVeSMSuSecRwLtStHPassStUpwdDnwdPosV_Val_read,IfVeSMSuSecRwLtStLgrstUpwdDnwdPosV_Val_read,IfVeSMSuSecRwLtStLtwdRtwdPosV_Val_read,IfVeSMSuSecRwLtStArmScrnPosV_Val_read
  Bus Selector5 : BusSelector  OutputSignals=IfVeSMSuSecRwLtStLgrstOtwdInwdPos_Val_read,IfVeSMSuRrLtStFtUpwdDnwdPos_Val_read,IfVeSMSuSecRwLtStHdrstFrwdBkwdPos_Val_read
  Bus Selector6 : BusSelector  OutputSignals=IfVeSMSuSecRwLtStLgrstOtwdInwdPosV_Val_read,IfVeSMSuRrLtStFtUpwdDnwdPosV_Val_read,IfVeSMSuSecRwLtStHdrstFrwdBkwdPosV_Val_read
  Bus Selector7 : BusSelector  OutputSignals=LyLSecRwLtSt.HdrstFrwdBkwdnwdPos,LyLSecRwLtSt.HdrstUpwdPos
  Chart : Stateflow chart  TreatAsAtomicUnit=on
  Chart1 : Stateflow chart  TreatAsAtomicUnit=on
  Logical Operator : Logic  Inputs=4  AllPortsSameDT=off  OutDataTypeStr=boolean
  Logical Operator1 : Logic  Inputs=3  AllPortsSameDT=off  OutDataTypeStr=boolean
  Logical Operator2 : Logic  AllPortsSameDT=off  OutDataTypeStr=boolean
  Logical Operator3 : Logic  AllPortsSameDT=off  OutDataTypeStr=boolean
  Logical Operator4 : Logic  Operator=NOT  AllPortsSameDT=off  OutDataTypeStr=boolean
  Logical Operator5 : Logic  AllPortsSameDT=off  OutDataTypeStr=boolean
  Logical Operator{6..9} (4 alike) : Logic  Operator=OR  AllPortsSameDT=off  OutDataTypeStr=boolean
  PA_KeSMSw4SSecRwLtStLgrstUpwdDnwdOpenPos1_Val : Constant  Value=KeSMSw4SSecRwLtStLgrstUpwdDnwdOpenPos1_Val
  R2Lt : Subsystem
  Relational Operator : RelationalOperator  OutDataTypeStr=boolean  RndMeth=Simplest
  Relational Operator1 : RelationalOperator  Operator=<  OutDataTypeStr=boolean  RndMeth=Simplest
  Relational Operator2 : RelationalOperator  Operator=<  OutDataTypeStr=boolean  RndMeth=Simplest
  Unit Delay1 : UnitDelay  SampleTime=-1
  Unit Delay3 : UnitDelay  SampleTime=-1
  Unit Delay4 : UnitDelay  SampleTime=-1
  VIP_TrigJudg : Lib/VIP_TrigJudg  SystemSampleTime=-1
  R2Lt_TrgtPoss : Outport  VectorParamsAs1DForOutWhenUnconnected=on
  IfVeSMSuSecRwLtStRclCmdSrv_Val_writeRec : Outport  Port=2
  isAcsMdFeedBackNew_LyL : Outport  Port=3
  R2Lt_TrgtPoss_2 : Outport  Port=4  VectorParamsAs1DForOutWhenUnconnected=on
  wires:
  R2Lt/4(IfVeSMSuSecRwLtStRclCmdSrv_Val_writeRaw) -> [IfVeSMSuSecRwLtStRclCmdSrv_Val_writeRaw]
  [IfVeSMSuSecRwLtStRclCmdSrv_Val_writeRaw] -> Chart1/2(IfVeSMSuSecRwLtStRclCmdSrv_Val_writeRaw)
  Recovery_Mod_Left/1 -> [Recovery_Mod_Left]
  Logical Operator/1 -> Chart1/1(Left_Done)
  R2Lt/1(R2Lt_Bk_Ini) -> [R2LtST_BkHd_ini]
  [Step1_En] -> R2Lt/2(Step1En)
  VIP_TrigJudg/1 -> [EZE_TrigL]
  [EZE_TrigL] -> R2Lt/1(Mode_Trig)
  R2Lt/3(R2Lt_TrgtPoss) -> R2Lt_TrgtPoss/1
  SecRwLtStsPoss/1 -> [Pos], R2Lt/3(SecRwLtStsPoss)
  SecRwLtStPossV/1 -> R2Lt/4(SecRwLtStPossV), [PosV]
  SecRwRtStChldLkRsp_L/1 -> R2Lt/5(SecRwRtStChldLkRsp_L)
  R2Lt/2(R2Lt_Bk_done) -> [R2LtST_BkHd_done]
  [R2LtST_BkHd_ini] -> Chart/1(R2Lt_ini)
  [R2LtST_BkHd_done] -> Chart/2(R2Lt_done)
  Chart/1(R2Lt_En) -> [Step1_En]
  [Recv_L_DoneOK] -> Chart1/3(Md_L_DoneOkRaw)
  [Recv_L_DoneFailed] -> Chart1/4(Md_L_DoneFailedRaw)
  Chart1/2(Md_L_DoneOk) -> [Ly_L_DoneOK]
  Chart1/3(Md_L_DoneFailed) -> [Ly_L_DoneFailed]
  Chart1/1(IfVeSMSuSecRwLtStRclCmdSrv_Val_write) -> IfVeSMSuSecRwLtStRclCmdSrv_Val_writeRec/1  "IfVeSMSuSecRwLtStRclCmdSrv_Val_write"
  Bus Selector/2 -> [ModeStCalib_Pass]  "<Calib_Pass>"
  Bus Selector/5 -> [ModeStCalib_3L]  "<Calib_3L>"
  Bus Selector/3 -> [ModeStCalib_2L]  "<Calib_2L>"
  Bus Selector/1 -> [ModeStCalib_Drv]  "<Calib_Drv>"
  Bus Selector/6 -> [ModeStCalib_3R]  "<Calib_3R>"
  Bus Selector/4 -> [ModeStCalib_2R]  "<Calib_2R>"
  ModeStCalib/1 -> Bus Selector/1
  [ModeStCalib_2L4s] -> R2Lt/6(ModeStCalib_2L)
  [Recovery_Mod_Left] -> VIP_TrigJudg/1
  Bus Creator1/1 -> isAcsMdFeedBackNew_LyL/1
  [Ly_L_DoneOK] -> Bus Creator1/1  "isLfLyDoneOK"
  [Ly_L_DoneFailed] -> Bus Creator1/2  "isLfLyDoneFailed"
  Bus Selector1/6 -> [ThdRwRtStConfig]  "<ThdRwRtStConfig>"
  Bus Selector1/1 -> [DrvStConfig]  "<DrvStConfig>"
  Bus Selector1/3 -> [SecRwLtStConfig]  "<SecRwLtStConfig>"
  Bus Selector1/4 -> [SecRwRtStConfig]  "<SecRwRtStConfig>"
  StConfig/1 -> Bus Selector1/1
  Bus Selector1/2 -> [PassStConfig]  "<PassStConfig>"
  Bus Selector1/5 -> [ThdRwLtStConfig]  "<ThdRwLtStConfig>"
  [SecRwLtStConfig] -> R2Lt/7(StConfig)
  Bus Selector/8 -> [ModeStCalib_2R4s]  "<Calib_2R4s>"
  Bus Selector/7 -> [ModeStCalib_2L4s]  "<Calib_2L4s>"
  SecRwLtStsPoss4s/1 -> [Pos4s], R2Lt/8(SecRwLtStsPoss4s)
  SecRwLtStPossV4s/1 -> R2Lt/9(SecRwLtStPossV4s), [PosV4s]
  StConfig4s/1 -> Bus Selector2/1
  Bus Selector2/1 -> [SecRwLtStConfig4s]  "<SecRwLtStConfig>"
  Bus Selector2/2 -> [SecRwRtStConfig4s]  "<SecRwRtStConfig>"
  [SecRwLtStConfig4s] -> R2Lt/10(StConfig4s)
  [PosV] -> Bus Selector4/1
  Bus Selector4/6 -> [R2LtStArmScrnPosV]  "<IfVeSMSuSecRwLtStArmScrnPosV_Val_read>"
  Bus Selector3/6 -> [R2LtStArmScrnPos]  "<IfVeSMSuSecRwLtStArmScrnPos_Val_read>"
  Bus Selector4/5 -> [SecRwLtStLtwdRtwdPosV]  "<IfVeSMSuSecRwLtStLtwdRtwdPosV_Val_read>"
  Bus Selector3/4 -> [SecRwLtStLgrstUpwdDnwdPos]  "<IfVeSMSuSecRwLtStLgrstUpwdDnwdPos_Val_read>"
  Bus Selector3/1 -> [SecRwLtStBkReclnUpwdDnwdPos]  "<IfVeSMSuSecRwLtStBkReclnUpwdDnwdPos_Val_read>"
  Bus Selector3/2 -> [SecRwLtStFrwdBkwdPos]  "<IfVeSMSuSecRwLtStFrwdBkwdPos_Val_read>"
  Bus Selector4/2 -> [SecRwLtStFrwdBkwdPosV]  "<IfVeSMSuSecRwLtStFrwdBkwdPosV_Val_read>"
  Bus Selector4/4 -> [SecRwLtStLgrstUpwdDnwdPosV]  "<IfVeSMSuSecRwLtStLgrstUpwdDnwdPosV_Val_read>"
  Bus Selector3/3 -> [SecRwLtStHPassStUpwdDnwdPos]  "<IfVeSMSuSecRwLtStHPassStUpwdDnwdPos_Val_read>"
  [Pos] -> Bus Selector3/1
  Bus Selector3/5 -> [SecRwLtStLtwdRtwdPos]  "<IfVeSMSuSecRwLtStLtwdRtwdPos_Val_read>"
  Bus Selector4/3 -> [SecRwLtStHPassStUpwdDnwdPosV]  "<IfVeSMSuSecRwLtStHPassStUpwdDnwdPosV_Val_read>"
  Bus Selector4/1 -> [SecRwLtStBkReclnUpwdDnwdPosV]  "<IfVeSMSuSecRwLtStBkReclnUpwdDnwdPosV_Val_read>"
  Bus Selector6/1 -> [SecRwLtStLgrstOtwdInwdPosV]  "<IfVeSMSuSecRwLtStLgrstOtwdInwdPosV_Val_read>"
  [Pos4s] -> Bus Selector5/1
  Bus Selector6/2 -> [RrLtStFtUpwdDnwdPosV]  "<IfVeSMSuRrLtStFtUpwdDnwdPosV_Val_read>"
  [PosV4s] -> Bus Selector6/1
  Bus Selector5/1 -> [SecRwLtStLgrstOtwdInwdPos]  "<IfVeSMSuSecRwLtStLgrstOtwdInwdPos_Val_read>"
  Bus Selector5/2 -> [RrLtStFtUpwdDnwdPos]  "<IfVeSMSuRrLtStFtUpwdDnwdPos_Val_read>"
  [SecRwLtStLgrstUpwdDnwdPos] -> Chart/3(pos)
  [StepEn_LgrstStep1] -> R2Lt/11(StepEn_LgrstStep1)
  [StepEn_LgrstStep2] -> R2Lt/12(StepEn_LgrstStep2)
  [StepEn_LgrstStep3] -> R2Lt/13(StepEn_LgrstStep3)
  R2Lt/5(lgrstStep1_ini) -> [lgrstStep1_ini]
  R2Lt/7(lgrstStep3_ini) -> [lgrstStep3_ini]
  R2Lt/6(lgrstStep2_ini) -> [lgrstStep2_ini]
  R2Lt/8(lgrstStep1_done) -> [lgrstStep1_done]
  R2Lt/10(lgrstStep3_done) -> [lgrstStep3_done]
  R2Lt/9(lgrstStep2_done) -> [lgrstStep2_done]
  [lgrstStep1_done] -> Chart/5(Step1done)
  [lgrstStep1_ini] -> Chart/8(Step1_ini)
  [lgrstStep2_ini] -> Chart/9(Step2_ini)
  [lgrstStep3_ini] -> Chart/10(Step3_ini)
  PA_KeSMSw4SSecRwLtStLgrstUpwdDnwdOpenPos1_Val/1 -> [OpenPos1]
  [OpenPos1] -> Chart/4(openpos1)
  Logical Operator2/1 -> Unit Delay1/1
  [lgrstStep3_done] -> Logical Operator3/1
  [SecRwLtStLgrstUpwdDnwdPos] -> Relational Operator/1
  [OpenPos1] -> Relational Operator/2
  Relational Operator/1 -> Unit Delay3/1
  [lgrstStep2_done] -> Logical Operator2/2
  Unit Delay1/1 -> [lgrstStep2_Chk], Chart/6(Step2done)
  Chart/2(StepEn_LgrstStep1) -> [StepEn_LgrstStep1]
  Chart/3(StepEn_LgrstStep2) -> [StepEn_LgrstStep2]
  Chart/4(StepEn_LgrstStep3) -> [StepEn_LgrstStep3]
  R2Lt/11(R2Lt_TrgtPoss_2) -> R2Lt_TrgtPoss_2/1
  Unit Delay3/1 -> Logical Operator2/1
  [lgrstStep2_Chk] -> Unit Delay4/1
  Logical Operator3/1 -> [lgrstStep3_Chk], Chart/7(Step3done)
  Unit Delay4/1 -> Logical Operator3/2
  Logical Operator4/1 -> [Recv_L_DoneFailed]
  isLfLyArrivedAtTargetPos/1 -> [Recv_L_DoneOK], Logical Operator4/1
  R2Lt/12(R2Lt_HdUp_Ini) -> [HdUp_ini]
  R2Lt/13(R2Lt_HdUp_Done) -> [HdUp_Done]
  R2Lt/14(R2Lt_HdFwd_Ini) -> [HFwd_ini]
  R2Lt/15(R2Lt_HdFwd_Done) -> [HFwd_Done]
  Bus Selector5/3 -> [SecRwLtStHdrstFrwdBkwdPos]  "<IfVeSMSuSecRwLtStHdrstFrwdBkwdPos_Val_read>"
  [SecRwLtStHdrstFrwdBkwdPos] -> Relational Operator1/1
  [SecRwLtStHPassStUpwdDnwdPos] -> Relational Operator2/1
  Relational Operator1/1 -> Logical Operator5/1
  Relational Operator2/1 -> Logical Operator5/2
  [ModeStCalib_2L4s] -> Bus Selector7/1
  Bus Selector7/1 -> Relational Operator1/2  "<HdrstFrwdBkwdnwdPos>"
  Bus Selector7/2 -> Relational Operator2/2  "<HdrstUpwdPos>"
  Chart/6(HdFwd_En) -> [HdFwd_En]
  Chart/5(HdUp_En) -> [HdUp_En]
  Logical Operator5/1 -> Chart/11(chkhdflg)
  [HdUp_Done] -> Chart/12(HdUp_Done)
  [HFwd_Done] -> Chart/13(HdFwd_Done)
  [HdUp_En] -> R2Lt/14(HdUp_En)
  [HdFwd_En] -> R2Lt/15(HdFwd_En)
  Chart/7(failflg) -> [failflg]
  Logical Operator1/1 -> Logical Operator6/1
  [failflg] -> Logical Operator6/2
  Logical Operator6/1 -> Logical Operator/1
  [HFwd_Done] -> Logical Operator/4
  [HdUp_Done] -> Logical Operator/3
  [R2LtST_BkHd_done] -> Logical Operator/2
  Bus Selector6/3 -> [SecRwLtStHdrstFrwdBkwdPosV]  "<IfVeSMSuSecRwLtStHdrstFrwdBkwdPosV_Val_read>"
  [lgrstStep1_done] -> Logical Operator7/1
  [lgrstStep1_ini] -> Logical Operator7/2
  [lgrstStep2_ini] -> Logical Operator8/2
  [lgrstStep2_Chk] -> Logical Operator8/1
  [lgrstStep3_Chk] -> Logical Operator9/1
  [lgrstStep3_ini] -> Logical Operator9/2
  Logical Operator9/1 -> Logical Operator1/3
  Logical Operator8/1 -> Logical Operator1/2
  Logical Operator7/1 -> Logical Operator1/1
  [HFwd_ini] -> Chart/15(HdFwd_ini)
  [HdUp_ini] -> Chart/14(HdUp_ini)
  Calib_Ly4sLAdpt/1 -> R2Lt/16(Calib_Ly4sLAdpt)
